simulink model "PrLiq2EE_PI_AntiWindup"  (R2022b)
settings: Solver=ode45  StartTime=0.0  StopTime=500  FixedStep=1  RelTol=1e-6  EnableMultiTasking=on
values from neighbouring files (symbols this model uses):
  a = k12/(2*Ar*sqrt(h1b-h2b))    [PrPara2nl_PI.m]    (also in para2nl.m; para2nl_PI.m)
  Ar = [0 0;1 0]    [PrObsPertContinuoRed.m]    (also in PrPara2nl_PI.m = 152.4; para2nl.m = 152.4; para2nl_PI.m = 152.4)
  b = k2/(2*Ar*sqrt(h2b))    [PrPara2nl_PI.m]    (also in para2nl.m; para2nl_PI.m)
  hmax = 16    [PrPara2nl_PI.m]    (also in para2nl.m; para2nl_PI.m)
  K = acker(A,B,p)    [PrObsPertContinuoRed.m]    (also in PrPara2nl_PI.m = acker(Aa,Ba,[p,p,p]); TestesEE.m = acker(A,B,[p,p,p]); TestesEEcanalI.m = acker(A,B,[p,-.6-1.0198i,-.6+1.0198i]); TestesEEobsPert.m = acker(A,B,[p,-.6-1.0198i,-.6+1.0198i]))
  k1 = 0    [PrPara2nl_PI.m]    (also in para2nl.m; para2nl_PI.m)
  k12 = 38    [PrPara2nl_PI.m]    (also in para2nl.m; para2nl_PI.m)
  k2 = 11.5    [PrPara2nl_PI.m]    (also in para2nl.m; para2nl_PI.m)
  Ki = -K(3)    [PrPara2nl_PI.m]    (also in TestesEEcanalI.m = -Ka(4),K=Ka(1:3),; para2nl_PI.m)
  Kp = -Ki/p    [PrPara2nl_PI.m]    (also in para2nl_PI.m)
  L = L'    [PrObsPertContinuoRed.m]    (also in PrPara2nl_PI.m; TestesEE.m; TestesEEcanalI.m; TestesEEobsPert.m)
  qmax = 90    [PrPara2nl_PI.m]    (also in para2nl.m; para2nl_PI.m)
  qmin = -85    [PrPara2nl_PI.m]    (also in para2nl.m; para2nl_PI.m)
libraries: simulink x1
settings Model: Creator=Adolfo  LastModifiedBy=adolfo
settings SolverCC: ZeroCrossControl=DisableAll  AlgebraicLoopSolver=TrustRegion
settings DataIOCC: LimitDataPoints=on  SaveFormat=Array  SignalLoggingSaveFormat=ModelDataLogs  ReturnWorkspaceOutputs=off
settings OptimizationCC: ExpressionDepthLimit=2147483647  InitFltsAndDblsToZero=on  LifeSpan=inf
settings DebuggingCC: SaveWithParameterizedLinksMsg=none  UnderspecifiedInitializationDetection=Classic  MergeDetectMultiDrivingBlocksExec=none  SignalResolutionControl=TryResolveAllWithWarning  SolverPrmCheckMsg=warning  MultiTaskDSMMsg=warning  MultiTaskCondExecSysMsg=none  FcnCallInpInsideContextMsg=warning  UnconnectedInputMsg=warning  UnconnectedOutputMsg=warning  UnconnectedLineMsg=warning  StateNameClashWarn=warning  SFUnexpectedBacktrackingDiag=warning  SFNoUnconditionalDefaultTransitionDiag=warning  SFExecutionAtInitializationDiag=none  SFMachineParentedDataDiag=warning  ArithmeticOperatorsInVariantConditions=warning
settings HardwareCC: ProdBitPerPointer=32  ProdBitPerSizeT=32  ProdBitPerPtrDiffT=32  ProdLargestAtomicFloat=None  ProdIntDivRoundTo=Undefined  ProdEndianess=Unspecified  ProdWordSize=32  ProdHWDeviceType=32-bit Generic
settings ModelReferenceCC: PropagateSignalLabelsOutOfModel=off
settings SFSimCC: SimUseLocalCustomCode=off  CustomCodeUndefinedFunction=UseInterfaceOnly
settings RTWCC: RTWUseLocalCustomCode=off
settings CodeAppCC: StateflowObjectComments=on
settings GRTTargetCC: TargetFcnLib=ansi_tfl_tmw.mat  TargetLangStandard=C89/C90 (ANSI)  CombineOutputUpdateFcns=off  GRTInterface=on
settings ConfigComp: CovMetricSettings=dw  CovSaveCumulativeToWorkspaceVar=on  CovSaveSingleToWorkspaceVar=on  CovExternalEMLEnable=off

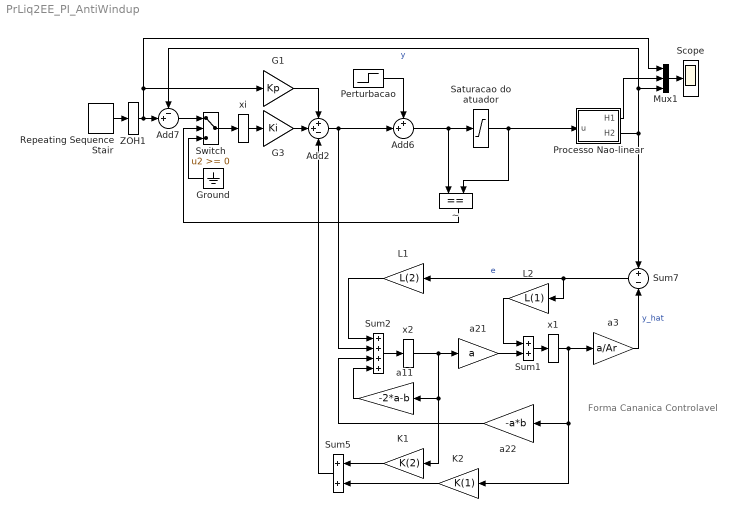
== system PrLiq2EE_PI_AntiWindup ==
  note: Forma
      | Cananica
      | Controlavel
  Add2 : Sum  Inputs=++-
  Add6 : Sum  Inputs=++|
  Add7 : Sum  Inputs=-+|
  G1 : Gain  Gain=Kp
  G3 : Gain  Gain=Ki
  Ground : Ground
  K1 : Gain  Gain=K(2)  SaturateOnIntegerOverflow=on  OutDataTypeStr=Inherit: Same as input  ParamDataTypeStr=Inherit: Same as input
  K2 : Gain  Gain=K(1)  SaturateOnIntegerOverflow=on  OutDataTypeStr=Inherit: Same as input  ParamDataTypeStr=Inherit: Same as input
  L1 : Gain  Gain=L(2)  SaturateOnIntegerOverflow=on  OutDataTypeStr=Inherit: Same as input  ParamDataTypeStr=Inherit: Same as input
  L2 : Gain  Gain=L(1)  SaturateOnIntegerOverflow=on  OutDataTypeStr=Inherit: Same as input  ParamDataTypeStr=Inherit: Same as input
  Mux1 : Mux  Inputs=3
  Perturbacao : Step  Time=350  After=200  SampleTime=0
  Processo Nao-linear : Subsystem
  Repeating Sequence Stair : simulink/Sources/Repeating Sequence Stair  OutValues=[2 5 12 5 2].'  tsamp=100  OutMin=[]  OutMax=[]  OutDataTypeStr=double  OutputDataTypeScalingMode=double  OutDataType=fixdt(0,8)  ConRadixGroup=Best Precision: Vector-wise  OutScaling=2^-12
  Saturacao do atuador : Saturate  UpperLimit=qmax  LowerLimit=qmin
  Scope : Scope
  Sum1 : Sum  InputSameDT=on  SaturateOnIntegerOverflow=on  OutDataTypeStr=Inherit: Same as first input
  Sum2 : Sum  Inputs=++++  InputSameDT=on  SaturateOnIntegerOverflow=on  OutDataTypeStr=Inherit: Same as first input
  Sum5 : Sum  InputSameDT=on  SaturateOnIntegerOverflow=on  OutDataTypeStr=Inherit: Same as first input
  Sum7 : Sum  Inputs=+-  InputSameDT=on  SaturateOnIntegerOverflow=on  OutDataTypeStr=Inherit: Same as first input
  Switch : Switch  OutDataTypeStr=Inherit: Inherit via back propagation  SaturateOnIntegerOverflow=off  InputSameDT=off
  ZOH1 : ZeroOrderHold
  a11 : Gain  Gain=-2*a-b  SaturateOnIntegerOverflow=on  OutDataTypeStr=Inherit: Same as input  ParamDataTypeStr=Inherit: Same as input
  a21 : Gain  Gain=a  SaturateOnIntegerOverflow=on  OutDataTypeStr=Inherit: Same as input  ParamDataTypeStr=Inherit: Same as input
  a22 : Gain  Gain=-a*b  SaturateOnIntegerOverflow=on  OutDataTypeStr=Inherit: Same as input  ParamDataTypeStr=Inherit: Same as input
  a3 : Gain  Gain=a/Ar  SaturateOnIntegerOverflow=on  OutDataTypeStr=Inherit: Same as input  ParamDataTypeStr=Inherit: Same as input
  x1 : Integrator
  x2 : Integrator
  xi : Integrator
  ~ : RelationalOperator  Operator===  OutDataTypeStr=boolean  InputSameDT=off
  wires:
  Mux1/1 -> Scope/1
  x2/1 -> a21/1, a11/1, K1/1
  Sum2/1 -> x2/1
  x1/1 -> a22/1, K2/1, a3/1
  Sum1/1 -> x1/1
  Add2/1 -> Sum2/2, Add6/2
  Processo Nao-linear/2(H2) -> Sum7/1, Mux1/3, Add7/1  "y"
  L1/1 -> Sum2/1
  K1/1 -> Sum5/1
  K2/1 -> Sum5/2
  Sum7/1 -> L1/1, L2/1  "e"
  a11/1 -> Sum2/4
  a22/1 -> Sum2/3
  a3/1 -> Sum7/2  "y_hat"
  Processo Nao-linear/1(H1) -> Mux1/2
  a21/1 -> Sum1/2
  L2/1 -> Sum1/1
  Perturbacao/1 -> Add6/1
  Add6/1 -> Saturacao do atuador/1, ~/1
  xi/1 -> G3/1
  Sum5/1 -> Add2/3
  G3/1 -> Add2/2
  G1/1 -> Add2/1
  Repeating Sequence Stair/1 -> ZOH1/1
  ZOH1/1 -> G1/1, Mux1/1, Add7/2
  Saturacao do atuador/1 -> Processo Nao-linear/1(u), ~/2
  Switch/1 -> xi/1
  Ground/1 -> Switch/3
  Add7/1 -> Switch/1
  ~/1 -> Switch/2

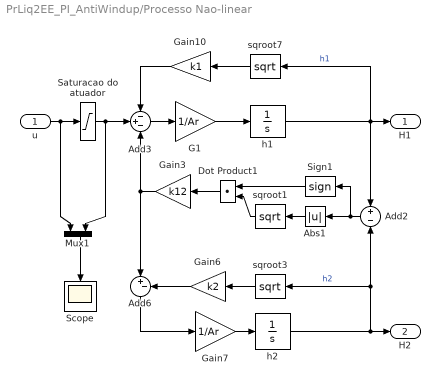
== system PrLiq2EE_PI_AntiWindup/Processo Nao-linear ==
  u : Inport
  Abs1 : Abs  SaturateOnIntegerOverflow=off
  Add2 : Sum  Inputs=+-
  Add3 : Sum  Inputs=-+-
  Add6 : Sum  Inputs=|+-
  Dot Product1 : DotProduct  OutDataTypeStr=Inherit: Inherit via internal rule
  G1 : Gain  Gain=1/Ar
  Gain10 : Gain  Gain=k1
  Gain3 : Gain  Gain=k12
  Gain6 : Gain  Gain=k2
  Gain7 : Gain  Gain=1/Ar
  Mux1 : Mux  Inputs=2
  Saturacao do atuador : Saturate  UpperLimit=qmax  LowerLimit=qmin
  Scope : Scope
  Sign1 : Signum
  h1 : Integrator  LimitOutput=on  UpperSaturationLimit=hmax  LowerSaturationLimit=0
  h2 : Integrator  LimitOutput=on  UpperSaturationLimit=hmax  LowerSaturationLimit=0
  sqroot1 : Math  Operator=sqrt  SignedPower=on
  sqroot3 : Math  Operator=sqrt  SignedPower=on
  sqroot7 : Math  Operator=sqrt  SignedPower=on
  H1 : Outport
  H2 : Outport  Port=2
  wires:
  h1/1 -> Add2/1, H1/1, sqroot7/1  "h1"
  h2/1 -> Add2/2, sqroot3/1, H2/1  "h2"
  Saturacao do atuador/1 -> Add3/2, Mux1/2
  Add6/1 -> Gain7/1
  Gain10/1 -> Add3/1
  sqroot7/1 -> Gain10/1
  Gain6/1 -> Add6/2
  Gain7/1 -> h2/1
  sqroot3/1 -> Gain6/1
  G1/1 -> h1/1
  Gain3/1 -> Add6/1, Add3/3
  Add3/1 -> G1/1
  Dot Product1/1 -> Gain3/1
  sqroot1/1 -> Dot Product1/2
  Sign1/1 -> Dot Product1/1
  Abs1/1 -> sqroot1/1
  Add2/1 -> Abs1/1, Sign1/1
  u/1 -> Saturacao do atuador/1, Mux1/1
  Mux1/1 -> Scope/1
